simulink model "winter_simulink_extremum_seeking_control"  (R2022a)
settings: Solver=FixedStepAuto  StartTime=0.0  StopTime=stop_time  FixedStep=1e-4  RelTol=1e-3
values from neighbouring files (symbols this model uses):
  B_eq = param{6}    [measurement_2states.m]    (also in measurement_2states_3mes.m; measurement_3measure.m)
  rho = param{2}    [measurement_3measure.m]
undefined symbols (not defined in the file or in its folder): blade, Gc, gearbox, generator, I_eq, lambda_vector, lookup_cP, omega_rated, pitch_range, pitch_vector, rotor, T_R0, wind
settings Model: Creator=Niccolò  LastModifiedBy=Niccolò

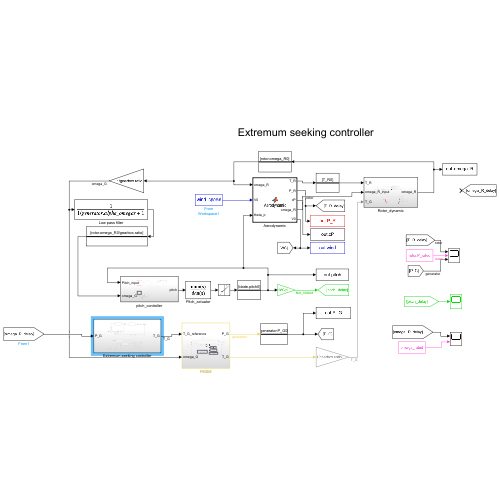
[thumbnail: Simulink's stored preview of the top-level diagram]
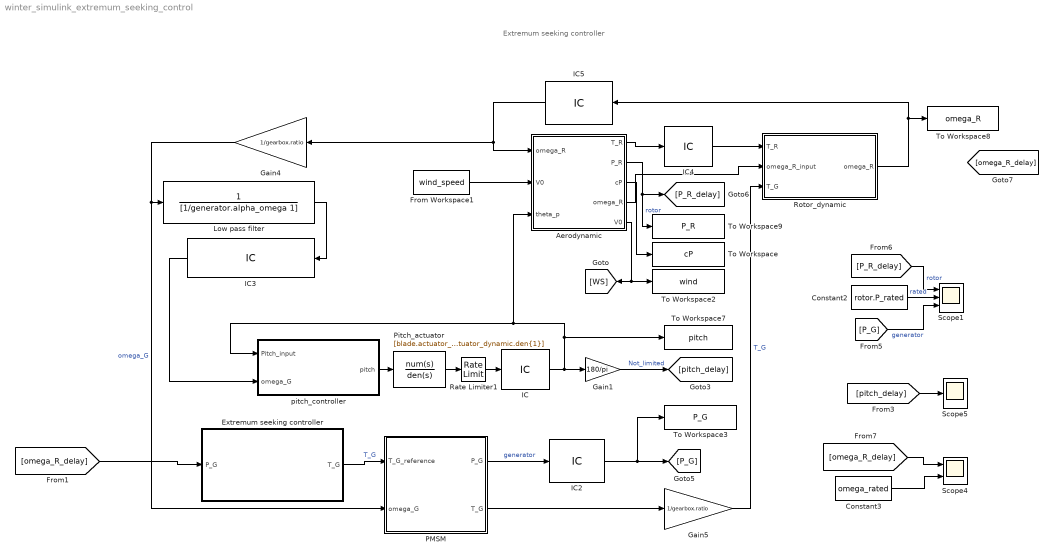
== system winter_simulink_extremum_seeking_control ==
  note: Extremum seeking controller
  Aerodynamic : MATLAB Function  TreatAsAtomicUnit=on
  Constant2 : Constant  Value=rotor.P_rated
  Constant3 : Constant  Value=omega_rated
  Extremum seeking controller : Subsystem
  From Workspace1 : FromWorkspace  VariableName=wind_speed  SampleTime=1/wind.sample_f
  Gain1 : Gain  Gain=180/pi
  Gain4 : Gain  Gain=1/gearbox.ratio
  Gain5 : Gain  Gain=1/gearbox.ratio
  IC : InitialCondition  Value=blade.pitch0
  IC2 : InitialCondition  Value=generator.P_G0
  IC3 : InitialCondition  Value=rotor.omega_R0/gearbox.ratio
  IC4 : InitialCondition  Value=T_R0
  IC5 : InitialCondition  Value=rotor.omega_R0
  Low pass filter : TransferFcn  Denominator=[1/generator.alpha_omega 1]
  PMSM : Subsystem
  Pitch_actuator : TransferFcn  Numerator=[blade.actuator_dynamic.num{1}]  Denominator=[blade.actuator_dynamic.den{1}]
  Rate Limiter1 : RateLimiter  RisingSlewLimit=blade.pitch_rate  FallingSlewLimit=-blade.pitch_rate  SampleTimeMode=inherited
  Rotor_dynamic : Subsystem
  Scope1 : Scope  NumInputPorts=3
  Scope4 : Scope  NumInputPorts=2
  Scope5 : Scope
  To Workspace : ToWorkspace  VariableName=cP  SaveFormat=Timeseries  SampleTime=-1
  To Workspace2 : ToWorkspace  VariableName=wind  SaveFormat=Timeseries  SampleTime=-1
  To Workspace3 : ToWorkspace  VariableName=P_G  SaveFormat=Timeseries  SampleTime=-1
  To Workspace7 : ToWorkspace  VariableName=pitch  SaveFormat=Timeseries  SampleTime=-1
  To Workspace8 : ToWorkspace  VariableName=omega_R  SaveFormat=Timeseries  SampleTime=-1
  To Workspace9 : ToWorkspace  VariableName=P_R  SaveFormat=Timeseries  SampleTime=-1
  pitch_controller : Subsystem
  wires:
  Rotor_dynamic/1(omega_R) -> IC5/1, To Workspace8/1
  Aerodynamic/5(V0) -> To Workspace2/1, [WS]
  IC5/1 -> Aerodynamic/1("omega_R "), Gain4/1
  Aerodynamic/3(cP) -> To Workspace/1
  Extremum seeking controller/1(T_G) -> PMSM/1(T_G_reference)  "T_G"
  Pitch_actuator/1 -> Rate Limiter1/1
  IC2/1 -> To Workspace3/1, [P_G]
  Aerodynamic/4(omega_R) -> Rotor_dynamic/2(omega_R_input)
  Aerodynamic/2(P_R) -> To Workspace9/1, [P_R_delay]  "rotor"
  pitch_controller/1(pitch) -> Pitch_actuator/1
  IC/1 -> Gain1/1, To Workspace7/1, Aerodynamic/3(theta_p), pitch_controller/1(Pitch_input)
  [pitch_delay] -> Scope5/1
  IC4/1 -> Rotor_dynamic/1(T_R)
  [P_G] -> Scope1/3  "generator"
  From Workspace1/1 -> Aerodynamic/2("V0 ")
  Gain5/1 -> Rotor_dynamic/3(T_G)  "T_G"
  Constant3/1 -> Scope4/2
  IC3/1 -> pitch_controller/2(omega_G)
  Gain1/1 -> [pitch_delay]  "Not_limited"
  PMSM/2(T_G) -> Gain5/1
  Constant2/1 -> Scope1/2  "rated"
  Low pass filter/1 -> IC3/1
  [P_R_delay] -> Scope1/1  "rotor"
  PMSM/1(P_G) -> IC2/1  "generator"
  Aerodynamic/1(T_R) -> IC4/1
  Gain4/1 -> PMSM/2(omega_G), Low pass filter/1  "omega_G"
  [omega_R_delay] -> Scope4/1
  Rate Limiter1/1 -> IC/1
  [omega_R_delay] -> Extremum seeking controller/1(P_G)

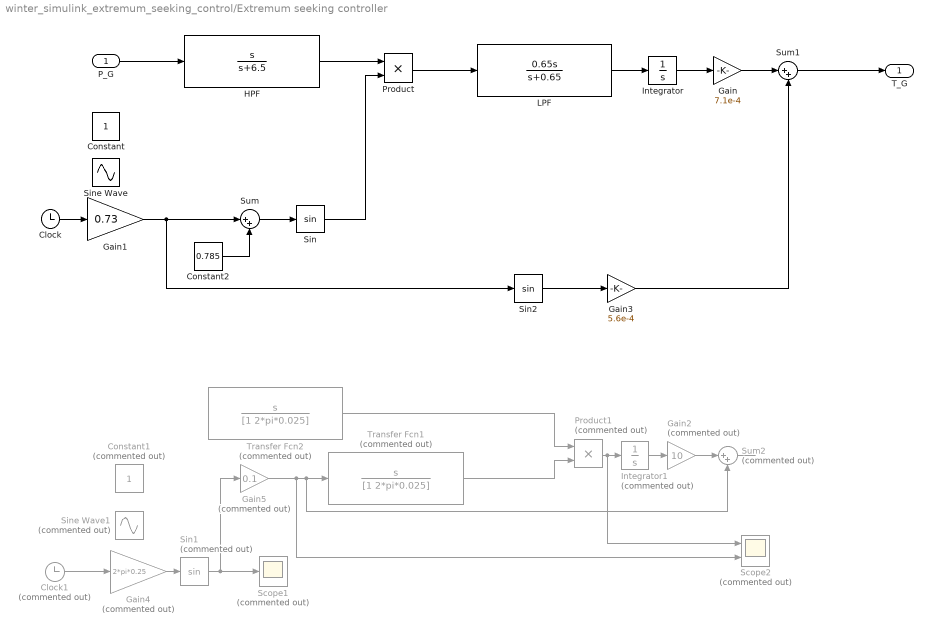
== system winter_simulink_extremum_seeking_control/Extremum seeking controller ==
  P_G : Inport
  Clock : Clock
  Clock1 : Clock  Commented=on
  Constant : Constant
  Constant1 : Constant  Commented=on
  Constant2 : Constant  Value=0.785
  Gain : Gain  Gain=7.1e-4
  Gain1 : Gain  Gain=0.73
  Gain2 : Gain  Commented=on  Gain=10
  Gain3 : Gain  Gain=5.6e-4
  Gain4 : Gain  Commented=on  Gain=2*pi*0.25
  Gain5 : Gain  Commented=on  Gain=0.1
  HPF : TransferFcn  Numerator=[1 0]  Denominator=[1 6.5]
  Integrator : Integrator
  Integrator1 : Integrator  Commented=on
  LPF : TransferFcn  Numerator=[0.65 0]  Denominator=[1 0.65]
  Product : Product
  Product1 : Product  Commented=on
  Scope1 : Scope  Commented=on
  Scope2 : Scope  Commented=on  NumInputPorts=2
  Sin : Trigonometry
  Sin1 : Trigonometry  Commented=on
  Sin2 : Trigonometry
  Sine Wave : Sin  Frequency=2*pi*0.25  SampleTime=0
  Sine Wave1 : Sin  Commented=on  Frequency=2*pi*0.25  SampleTime=0
  Sum : Sum  Inputs=|++
  Sum1 : Sum  Inputs=|++
  Sum2 : Sum  Commented=on  Inputs=|++
  Transfer Fcn1 : TransferFcn  Commented=on  Numerator=[1 0]  Denominator=[1 2*pi*0.025]
  Transfer Fcn2 : TransferFcn  Commented=on  Numerator=[1 0]  Denominator=[1 2*pi*0.025]
  T_G : Outport
  wires:
  Integrator/1 -> Gain/1
  P_G/1 -> HPF/1
  Gain/1 -> Sum1/1
  Product/1 -> LPF/1
  HPF/1 -> Product/1
  Sum1/1 -> T_G/1
  Clock/1 -> Gain1/1
  Clock1/1 -> Gain4/1
  Sum2/1 -> ?
  Product1/1 -> Scope2/1, Integrator1/1
  Gain2/1 -> Sum2/1
  ? -> Transfer Fcn2/1
  Transfer Fcn1/1 -> Product1/2
  Integrator1/1 -> Gain2/1
  Gain5/1 -> Transfer Fcn1/1, Sum2/2, Scope2/2
  Sin1/1 -> Scope1/1, Gain5/1
  Transfer Fcn2/1 -> Product1/1
  Gain4/1 -> Sin1/1
  Gain1/1 -> Sum/1, Sin2/1
  Sum/1 -> Sin/1
  Constant2/1 -> Sum/2
  Sin/1 -> Product/2
  LPF/1 -> Integrator/1
  Sin2/1 -> Gain3/1
  Gain3/1 -> Sum1/2

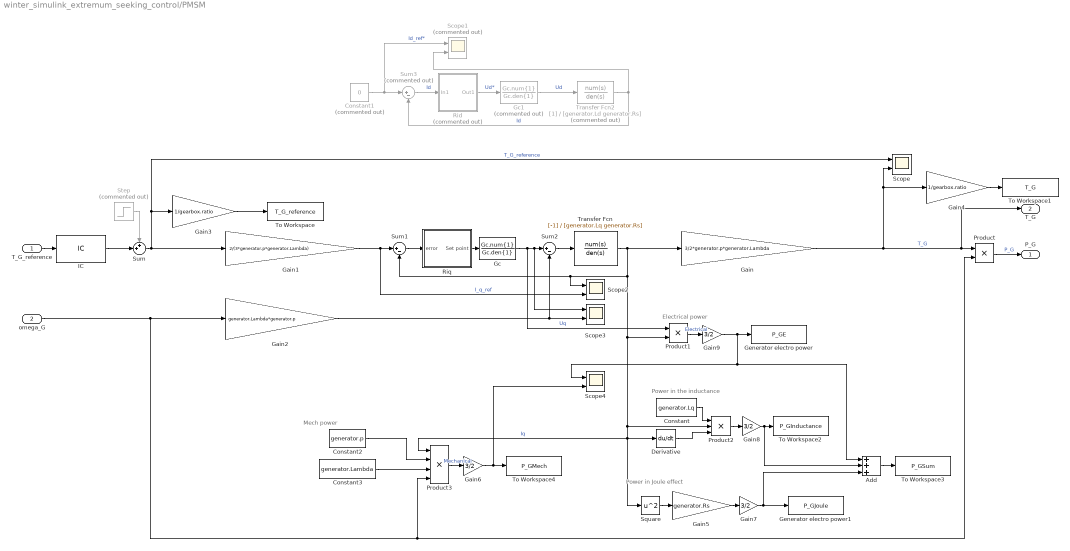
== system winter_simulink_extremum_seeking_control/PMSM ==
  note: Power in Joule effect
  note: Power in the inductance
  note: Electrical power
  note: Mech power
  T_G_reference : Inport
  omega_G : Inport  Port=2
  Add : Sum  Inputs=3
  Constant : Constant  Value=generator.Lq
  Constant1 : Constant  Commented=on  Value=0
  Constant2 : Constant  Value=generator.p
  Constant3 : Constant  Value=generator.Lambda
  Derivative : Derivative
  Gain : Gain  Gain=3/2*generator.p*generator.Lambda
  Gain1 : Gain  Gain=2/(3*generator.p*generator.Lambda)
  Gain2 : Gain  Gain=generator.Lambda*generator.p
  Gain3 : Gain  Gain=1/gearbox.ratio
  Gain4 : Gain  Gain=1/gearbox.ratio
  Gain5 : Gain  Gain=generator.Rs
  Gain{6..9} (4 alike) : Gain  Gain=3/2
  Gc : TransferFcn  Numerator=Gc.num{1}  Denominator=Gc.den{1}
  Gc1 : TransferFcn  Commented=on  Numerator=Gc.num{1}  Denominator=Gc.den{1}
  Generator electro power : ToWorkspace  VariableName=P_GE  SaveFormat=Timeseries  SampleTime=-1
  Generator electro power1 : ToWorkspace  VariableName=P_GJoule  SaveFormat=Timeseries  SampleTime=-1
  IC : InitialCondition  Value=generator.T_G0
  Product : Product
  Product1 : Product
  Product2 : Product  Inputs=3
  Product3 : Product  Inputs=4
  Rid : Subsystem  Commented=on
  Riq : Subsystem
  Scope{,2..4} (4 alike) : Scope  NumInputPorts=2
  Scope1 : Scope  Commented=on  NumInputPorts=2
  Square : Math  Operator=square
  Step : Step  Commented=on  Time=0.5  SampleTime=0
  Sum : Sum  Inputs=++|
  Sum1 : Sum  Inputs=|+-
  Sum2 : Sum  Inputs=|+-
  Sum3 : Sum  Commented=on  Inputs=|+-
  To Workspace : ToWorkspace  VariableName=T_G_reference  SaveFormat=Timeseries  SampleTime=-1
  To Workspace1 : ToWorkspace  VariableName=T_G  SaveFormat=Timeseries  SampleTime=-1
  To Workspace2 : ToWorkspace  VariableName=P_GInductance  SaveFormat=Timeseries  SampleTime=-1
  To Workspace3 : ToWorkspace  VariableName=P_GSum  SaveFormat=Timeseries  SampleTime=-1
  To Workspace4 : ToWorkspace  VariableName=P_GMech  SaveFormat=Timeseries  SampleTime=-1
  Transfer Fcn : TransferFcn  Numerator=[-1]  Denominator=[generator.Lq generator.Rs]
  Transfer Fcn2 : TransferFcn  Commented=on  Denominator=[generator.Ld generator.Rs]
  P_G : Outport
  T_G : Outport  Port=2
  wires:
  Gc/1 -> Product1/1, Scope3/1, Sum2/1  "Uq"
  Gain/1 -> T_G/1, Product/1, Gain4/1, Scope/2  "T_G"
  Riq/1(Set point) -> Gc/1
  Sum1/1 -> Riq/1(error)
  Transfer Fcn/1 -> Gain/1, Scope2/1, Sum1/2, Product1/2, Product3/1, Square/1, Derivative/1, Product2/2  "Iq"
  Product/1 -> P_G/1  "P_G"
  Gain1/1 -> Scope2/2, Sum1/1  "I_q_ref"
  Sum/1 -> Gain1/1, Scope/1, Gain3/1  "T_G_reference"
  T_G_reference/1 -> IC/1
  Step/1 -> Sum/1
  Sum2/1 -> Transfer Fcn/1
  Gain3/1 -> To Workspace/1
  IC/1 -> Sum/2
  Gain5/1 -> Gain7/1
  Square/1 -> Gain5/1
  Derivative/1 -> Product2/3
  Constant/1 -> Product2/1
  Product2/1 -> Gain8/1
  Gc1/1 -> Transfer Fcn2/1  "Ud"
  Rid/1(Out1) -> Gc1/1  "Ud*"
  Transfer Fcn2/1 -> Sum3/2, Scope1/2  "Id"
  Constant1/1 -> Scope1/1, Sum3/1  "Id_ref*"
  Sum3/1 -> Rid/1(In1)  "Id"
  Add/1 -> To Workspace3/1
  Constant2/1 -> Product3/2
  Constant3/1 -> Product3/3
  Product3/1 -> Gain6/1  "Mechanical"
  Product1/1 -> Gain9/1  "Electrical"
  Gain2/1 -> Scope3/2, Sum2/2
  omega_G/1 -> Product/2, Product3/4, Gain2/1
  Gain6/1 -> Scope4/2, To Workspace4/1
  Gain7/1 -> Generator electro power1/1, Add/3
  Gain8/1 -> To Workspace2/1, Add/2
  Gain9/1 -> Generator electro power/1, Add/1, Scope4/1
  Gain4/1 -> To Workspace1/1

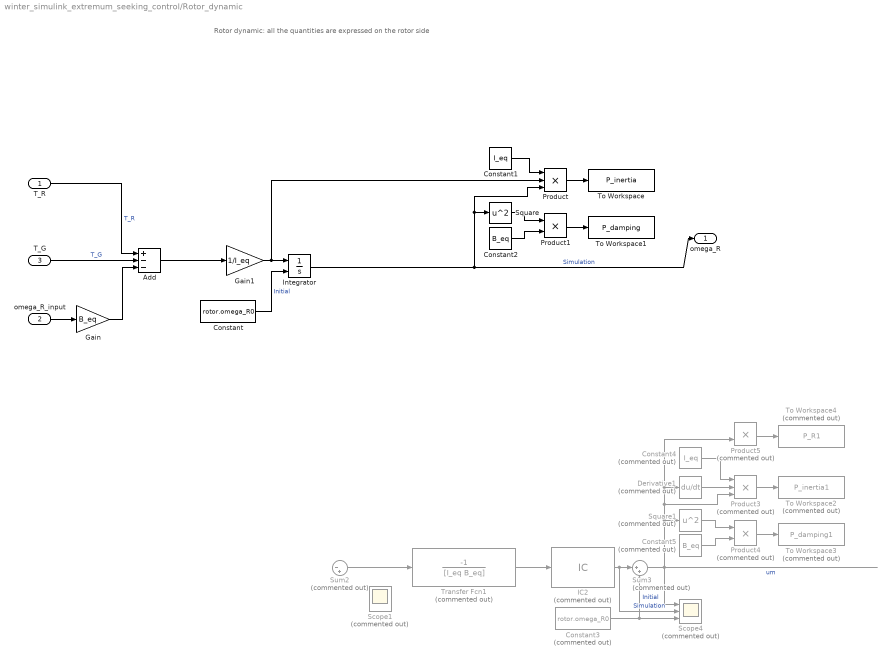
== system winter_simulink_extremum_seeking_control/Rotor_dynamic ==
  note: Rotor dynamic: all the quantities are expressed on the rotor side
  T_R : Inport
  omega_R_input : Inport  Port=2
  T_G : Inport  Port=3
  Add : Sum  Inputs=+--
  Constant : Constant  Value=rotor.omega_R0
  Constant1 : Constant  Value=I_eq
  Constant2 : Constant  Value=B_eq
  Constant3 : Constant  Commented=on  Value=rotor.omega_R0
  Constant4 : Constant  Commented=on  Value=I_eq
  Constant5 : Constant  Commented=on  Value=B_eq
  Derivative1 : Derivative  Commented=on
  Gain : Gain  Gain=B_eq
  Gain1 : Gain  Gain=1/I_eq
  IC2 : InitialCondition  Commented=on  Value=rotor.omega_R0
  Integrator : Integrator  InitialConditionSource=external
  Product : Product  Inputs=3
  Product1 : Product
  Product3 : Product  Commented=on  Inputs=3
  Product4 : Product  Commented=on
  Product5 : Product  Commented=on
  Scope1 : Scope  Commented=on  NumInputPorts=2
  Scope4 : Scope  Commented=on  NumInputPorts=3
  Square : Math  Operator=square
  Square1 : Math  Commented=on  Operator=square
  Sum2 : Sum  Commented=on  Inputs=|-+
  Sum3 : Sum  Commented=on  Inputs=|++
  To Workspace : ToWorkspace  VariableName=P_inertia  SaveFormat=Timeseries  SampleTime=-1
  To Workspace1 : ToWorkspace  VariableName=P_damping  SaveFormat=Timeseries  SampleTime=-1
  To Workspace2 : ToWorkspace  Commented=on  VariableName=P_inertia1  SaveFormat=Timeseries  SampleTime=-1
  To Workspace3 : ToWorkspace  Commented=on  VariableName=P_damping1  SaveFormat=Timeseries  SampleTime=-1
  To Workspace4 : ToWorkspace  Commented=on  VariableName=P_R1  SaveFormat=Timeseries  SampleTime=-1
  Transfer Fcn1 : TransferFcn  Commented=on  Numerator=[-1]  Denominator=[I_eq B_eq]
  omega_R : Outport
  wires:
  Integrator/1 -> Product/3, Square/1, omega_R/1  "Simulation"
  T_G/1 -> Add/2  "T_G"
  Constant/1 -> Integrator/2  "Initial"
  T_R/1 -> Add/1  "T_R"
  Add/1 -> Gain1/1
  Constant1/1 -> Product/1
  Product/1 -> To Workspace/1
  Constant2/1 -> Product1/2
  Product1/1 -> To Workspace1/1
  Square/1 -> Product1/1
  Square1/1 -> Product4/1
  Product5/1 -> To Workspace4/1
  Derivative1/1 -> Product3/2
  Product4/1 -> To Workspace3/1
  Constant4/1 -> Product3/1
  Constant5/1 -> Product4/2
  ? -> Scope1/2, Sum2/1, Product5/1  "T_R"
  ? -> Scope1/1, Sum2/2  "T_G"
  IC2/1 -> Scope4/2, Sum3/1  "Simulation"
  Sum2/1 -> Transfer Fcn1/1
  Product3/1 -> To Workspace2/1
  Transfer Fcn1/1 -> IC2/1
  Sum3/1 -> Product5/2, Derivative1/1, Product3/3, Square1/1, Scope4/1  "um"
  Constant3/1 -> Scope4/3, Sum3/2  "Initial"
  omega_R_input/1 -> Gain/1
  Gain/1 -> Add/3
  Gain1/1 -> Integrator/1, Product/2

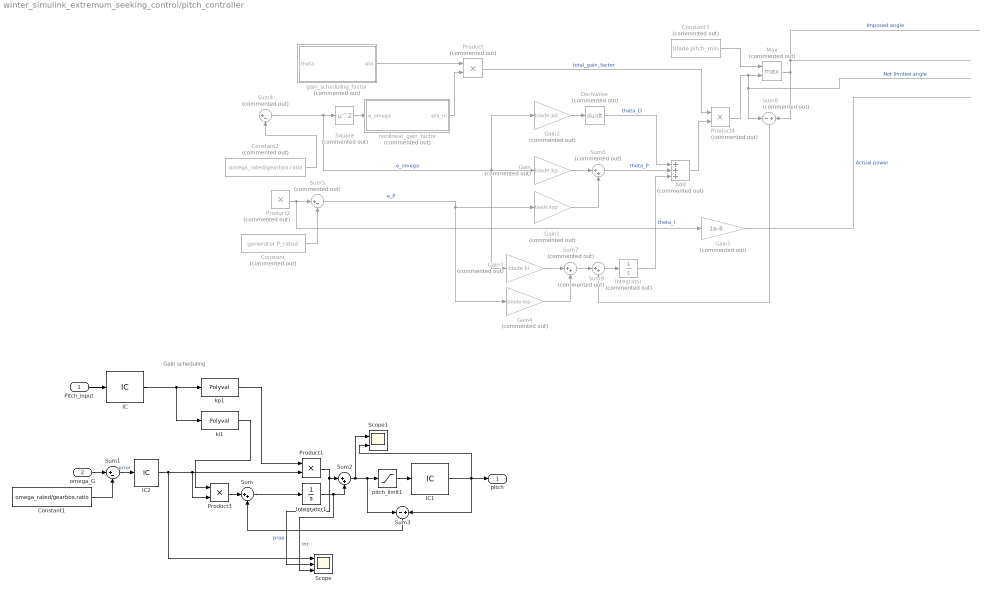
== system winter_simulink_extremum_seeking_control/pitch_controller ==
  note: Gain scheduling
  Pitch_input : Inport
  omega_G : Inport  Port=2
  Add : Sum  Commented=on  Inputs=+++
  Constant : Constant  Commented=on  Value=generator.P_rated
  Constant1 : Constant  Value=omega_rated/gearbox.ratio
  Constant2 : Constant  Commented=on  Value=omega_rated/gearbox.ratio
  Constant3 : Constant  Commented=on  Value=blade.pitch_min
  Derivative : Derivative  Commented=on
  Gain : Gain  Commented=on  Gain=blade.kp
  Gain1 : Gain  Commented=on  Gain=blade.kpp
  Gain2 : Gain  Commented=on  Gain=blade.kd
  Gain3 : Gain  Commented=on  Gain=blade.ki
  Gain4 : Gain  Commented=on  Gain=blade.kip
  Gain5 : Gain  Commented=on  Gain=1e-8
  IC : InitialCondition  Value=blade.pitch0
  IC1 : InitialCondition  Value=blade.pitch0
  IC2 : InitialCondition  Value=(rotor.omega_R0 - omega_rated)/gearbox.ratio
  Integrator : Integrator  Commented=on
  Integrator1 : Integrator
  Max : MinMax  Commented=on  Function=max  Inputs=2
  Product : Product  Commented=on
  Product1 : Product
  Product2 : Product  Commented=on
  Product3 : Product
  Product4 : Product  Commented=on
  Scope : Scope  NumInputPorts=3
  Scope1 : Scope  NumInputPorts=2
  Square : Math  Commented=on  Operator=square
  Sum : Sum  Inputs=|++
  Sum1 : Sum  Inputs=|+-
  Sum2 : Sum  Inputs=|++
  Sum3 : Sum  Inputs=-|+
  Sum4 : Sum  Commented=on  Inputs=|+-
  Sum5 : Sum  Commented=on  Inputs=|+-
  Sum6 : Sum  Commented=on  Inputs=|++
  Sum7 : Sum  Commented=on  Inputs=|++
  Sum8 : Sum  Commented=on  Inputs=-|+
  Sum9 : Sum  Commented=on  Inputs=|++
  gain_scheduling_factor : MATLAB Function  Commented=on  TreatAsAtomicUnit=on
  ki1 : Polyval  Coefs=blade.ki_schedule
  kp1 : Polyval  Coefs=blade.kp_schedule
  nonlinear_gain_factor : MATLAB Function  Commented=on  TreatAsAtomicUnit=on
  pitch_limit1 : Saturate  UpperLimit=pitch_range(2)  LowerLimit=0
  pitch : Outport
  wires:
  Sum/1 -> Integrator1/1
  Constant1/1 -> Sum1/2
  Product3/1 -> Sum/1
  omega_G/1 -> Sum1/1
  ki1/1 -> Product3/1
  kp1/1 -> Product1/1
  Sum1/1 -> IC2/1  "error"
  Product1/1 -> Scope/2, Sum2/1  "prop"
  Integrator1/1 -> Scope/3, Sum2/2  "int"
  ? -> ?  "Actual value"
  Sum8/1 -> Sum9/2
  Product4/1 -> Max/2, Sum8/1  "Not limited angle"
  Add/1 -> Product4/2
  Gain4/1 -> Sum7/2
  Product2/1 -> Gain5/1, Sum5/1
  Integrator/1 -> Add/3  "theta_I"
  ? -> Product2/2
  Derivative/1 -> Add/1  "theta_D"
  Product/1 -> Product4/1  "total_gain_factor"
  Sum6/1 -> Add/2  "theta_P"
  nonlinear_gain_factor/1(eta_nl) -> Product/2
  gain_scheduling_factor/1(eta) -> Product/1
  Gain/1 -> Sum6/1
  Max/1 -> Sum8/2  "Imposed angle"
  Sum5/1 -> Gain4/1, Gain1/1  "e_P"
  ? -> Sum4/1, Product2/1
  Constant2/1 -> Sum4/2
  Sum4/1 -> Gain3/1, Gain2/1, Gain/1, Square/1  "e_omega"
  Gain2/1 -> Derivative/1
  ? -> gain_scheduling_factor/1(theta)
  Gain5/1 -> ?  "Actual power"
  Constant/1 -> Sum5/2
  Constant3/1 -> Max/1
  Sum9/1 -> Integrator/1
  Gain1/1 -> Sum6/2
  Sum7/1 -> Sum9/1
  Square/1 -> nonlinear_gain_factor/1(e_omega)
  Gain3/1 -> Sum7/1
  Pitch_input/1 -> IC/1
  Sum2/1 -> pitch_limit1/1, Sum3/1, Scope1/1
  Sum3/1 -> Sum/2
  pitch_limit1/1 -> IC1/1
  IC/1 -> ki1/1, kp1/1
  IC1/1 -> Scope1/2, pitch/1, Sum3/2
  IC2/1 -> Scope/1, Product3/2, Product1/2

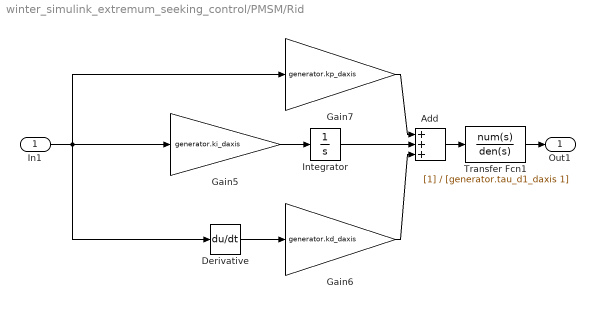
== system winter_simulink_extremum_seeking_control/PMSM/Rid ==
  In1 : Inport
  Add : Sum  Inputs=+++
  Derivative : Derivative
  Gain5 : Gain  Gain=generator.ki_daxis
  Gain6 : Gain  Gain=generator.kd_daxis
  Gain7 : Gain  Gain=generator.kp_daxis
  Integrator : Integrator
  Transfer Fcn1 : TransferFcn  Denominator=[generator.tau_d1_daxis 1]
  Out1 : Outport
  wires:
  Integrator/1 -> Add/2
  Add/1 -> Transfer Fcn1/1
  Gain7/1 -> Add/1
  Gain6/1 -> Add/3
  Derivative/1 -> Gain6/1
  In1/1 -> Derivative/1, Gain7/1, Gain5/1
  Transfer Fcn1/1 -> Out1/1
  Gain5/1 -> Integrator/1

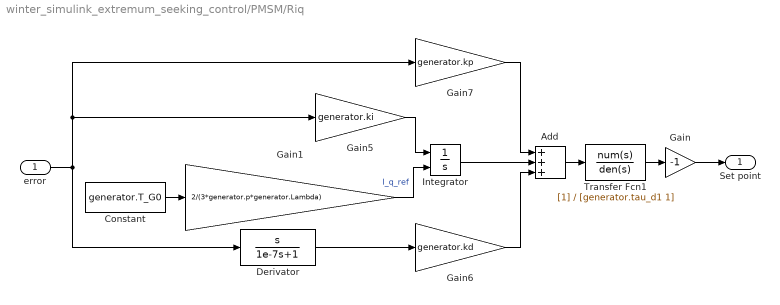
== system winter_simulink_extremum_seeking_control/PMSM/Riq ==
  error : Inport
  Add : Sum  Inputs=+++
  Constant : Constant  Value=generator.T_G0
  Derivator : TransferFcn  Numerator=[1 0]  Denominator=[1e-7 1]
  Gain : Gain  Gain=-1
  Gain1 : Gain  Gain=2/(3*generator.p*generator.Lambda)
  Gain5 : Gain  Gain=generator.ki
  Gain6 : Gain  Gain=generator.kd
  Gain7 : Gain  Gain=generator.kp
  Integrator : Integrator  InitialConditionSource=external
  Transfer Fcn1 : TransferFcn  Denominator=[generator.tau_d1 1]
  Set point : Outport
  wires:
  Integrator/1 -> Add/2
  Add/1 -> Transfer Fcn1/1
  Constant/1 -> Gain1/1
  Gain7/1 -> Add/1
  Gain6/1 -> Add/3
  Derivator/1 -> Gain6/1
  error/1 -> Gain5/1, Gain7/1, Derivator/1
  Transfer Fcn1/1 -> Gain/1
  Gain5/1 -> Integrator/1
  Gain1/1 -> Integrator/2  "I_q_ref"
  Gain/1 -> Set point/1

== matlab function winter_simulink_extremum_seeking_control/Aerodynamic ==
  data: omega_R input; V0 input; T_R output; P_R output; rho parameter; theta_p input; lambda_vector parameter; pitch_vector parameter; lookup_cP parameter; cP output; rotor parameter; omega_R output; V0 output
function [T_R, P_R, cP, omega_R, V0] = Aerodynamic(omega_R, V0, rho, theta_p, lambda_vector, pitch_vector, lookup_cP, rotor)

R = rotor.R;                  % rotor radius [m]

% retrive the cP from the look-up table
lambda = omega_R*R/V0;                                                
cP = interp2(lambda_vector, pitch_vector, lookup_cP, lambda, theta_p);

P_R = 0.5*rho*V0^3*pi*R^2*cP; % rotor power [W]
T_R = P_R/omega_R;            % rotor torque [Nm]

== matlab function winter_simulink_extremum_seeking_control/pitch_controller/gain_scheduling_factor ==
  data: eta output; theta input; blade parameter
function eta = gain_scheduling_factor(theta, blade)

K1 = blade.K1;
K2 = blade.K2;

theta = theta*180/pi; % [deg]

eta = 1/(1+ theta/K1 + theta^2/K2);

== matlab function winter_simulink_extremum_seeking_control/pitch_controller/nonlinear_gain_factor ==
  data: e_omega input; eta_nl output; blade parameter; generator parameter
function eta_nl = nonlinear_gain_factor(e_omega, blade, generator)

omega_rated = generator.omega_rated;
omega2 = omega_rated*blade.omega2omega0ratio;

eta_nl = 1 + e_omega^2/(omega2 - omega_rated)^2;
